simulink model "DevelopmentESP32_Centering"  (R2024b)
settings: Solver=FixedStepAuto  StartTime=0.0  StopTime=inf  RelTol=1e-3  EnableMultiTasking=on
libraries: arduinolib x2
(part 2 of 2)

== matlab function DevelopmentESP32_Centering/Map Function2 ==
  data: x input; y output; in_min input; in_max input; out_min input; data input; out_max input
function y = map(x,in_min,in_max,out_min,data, out_max)
    y = (x - in_min) * (out_max - out_min) / (in_max - in_min) + out_min;
end

== matlab function DevelopmentESP32_Centering/Map Function3 ==
  data: x input; y output; in_min input; in_max input; out_min input; data input; out_max input
function y = map(x,in_min,in_max,out_min,data, out_max)
    y = (x - in_min) * (out_max - out_min) / (in_max - in_min) + out_min;
end
